simulink model "prb3"  (R2020a)
settings: Solver=VariableStepAuto  StartTime=0.0  StopTime=10.0  RelTol=1e-3
settings Model: Creator=Riyansh  LastModifiedBy=Riyansh

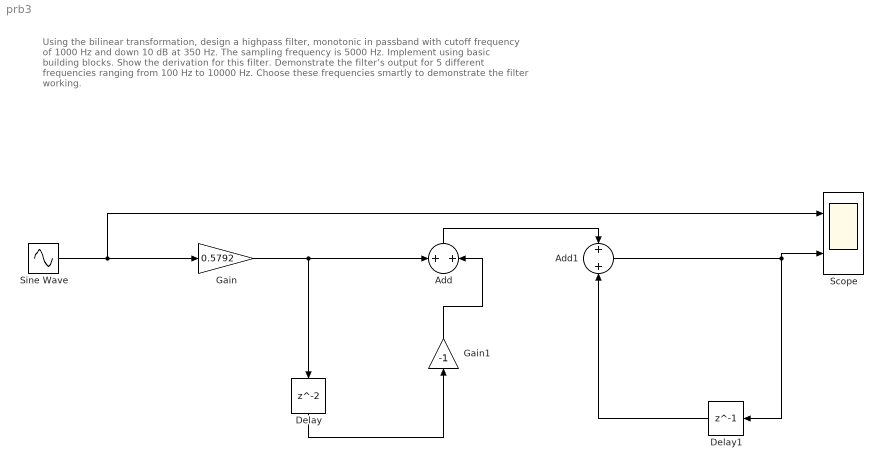
== system prb3 ==
  note: Using the bilinear transformation, design a highpass filter, monotonic in passband with cutoff frequency of 1000 Hz
      | and down 10 dB at 350 Hz. The sampling frequency is 5000 Hz. Implement using basic building blocks. Show the
      | derivation for this filter. Demonstrate the filter’s output for 5 different frequencies ranging from 100 Hz to 10000 Hz.
      | Choose these frequencies smartly to demonstrate the filter working.
  Add : Sum
  Add1 : Sum
  Delay : Delay
  Delay1 : Delay  DelayLength=1
  Gain : Gain  Gain=0.5792
  Gain1 : Gain  Gain=-1
  Scope : Scope  NumInputPorts=2
  Sine Wave : Sin  Phase=2e-10  SampleTime=0
  wires:
  Sine Wave/1 -> Scope/1, Gain/1
  Add1/1 -> Delay1/1, Scope/2
  Delay1/1 -> Add1/2
  Delay/1 -> Gain1/1
  Gain/1 -> Delay/1, Add/1
  Gain1/1 -> Add/2
  Add/1 -> Add1/1
